simulink model "nested"  (R2020b)
settings: Solver=ode45  StartTime=0.0  StopTime=250  RelTol=1e-3  EnableMultiTasking=on
values from neighbouring files (symbols this model uses):
  apsi1 = 2.374    [Principal.m]
  apsi2 = 0.08    [Principal.m]
  az1 = 3    [Principal.m]
  az2 = 0.5    [Principal.m]
  bphi1 = 2    [Principal.m]
  bphi2 = 1    [Principal.m]
  bphi3 = 0.2    [Principal.m]
  bphi4 = 0.1    [Principal.m]
  bth1 = 2    [Principal.m]
  bth2 = 1    [Principal.m]
  bth3 = 0.2    [Principal.m]
  bth4 = 0.1    [Principal.m]
  ci_phi = 0    [Principal.m]
  ci_phip = 0    [Principal.m]
  ci_psi = 0    [Principal.m]
  ci_psip = 0    [Principal.m]
  ci_th = 0    [Principal.m]
  ci_thp = 0    [Principal.m]
  ci_x = 100    [Principal.m]
  ci_xp = 0    [Principal.m]
  ci_y = 70    [Principal.m]
  ci_yp = 0    [Principal.m]
  ci_z = 0    [Principal.m]
  ci_zp = 0    [Principal.m]
  g = 9.81    [Principal.m]
  m = 0.52    [Principal.m]
  mg = m*g    (= 5.1012)    [Principal.m]
  psid = 0.5    [Principal.m]
  zd = 50    [Principal.m]
libraries: simulink x32
settings Model: Creator=cesar  LastModifiedBy=20808
settings DataIOCC: LimitDataPoints=on  SaveFormat=Array  SignalLoggingSaveFormat=ModelDataLogs  ReturnWorkspaceOutputs=off
settings OptimizationCC: ExpressionDepthLimit=2147483647  InitFltsAndDblsToZero=on  LifeSpan=inf
settings DebuggingCC: UnderspecifiedInitializationDetection=Classic  MergeDetectMultiDrivingBlocksExec=none  SolverPrmCheckMsg=warning  FcnCallInpInsideContextMsg=warning  StateNameClashWarn=warning  SFUnexpectedBacktrackingDiag=warning  SFNoUnconditionalDefaultTransitionDiag=warning  SFExecutionAtInitializationDiag=none  ArithmeticOperatorsInVariantConditions=warning
settings HardwareCC: ProdBitPerPointer=32  ProdBitPerSizeT=32  ProdBitPerPtrDiffT=32  ProdLargestAtomicFloat=None  ProdIntDivRoundTo=Undefined  ProdEndianess=Unspecified  ProdWordSize=32  ProdHWDeviceType=32-bit Generic
settings ModelReferenceCC: PropagateSignalLabelsOutOfModel=off
settings SFSimCC: SimUseLocalCustomCode=off  SimParseCustomCode=off  CustomCodeUndefinedFunction=UseInterfaceOnly
settings RTWCC: RTWUseLocalCustomCode=off
settings CodeAppCC: StateflowObjectComments=on
settings GRTTargetCC: TargetLangStandard=C89/C90 (ANSI)  CombineOutputUpdateFcns=off  GRTInterface=on
settings ConfigComp: CovMetricSettings=dw  CovSaveCumulativeToWorkspaceVar=on  CovSaveSingleToWorkspaceVar=on  CovExternalEMLEnable=off

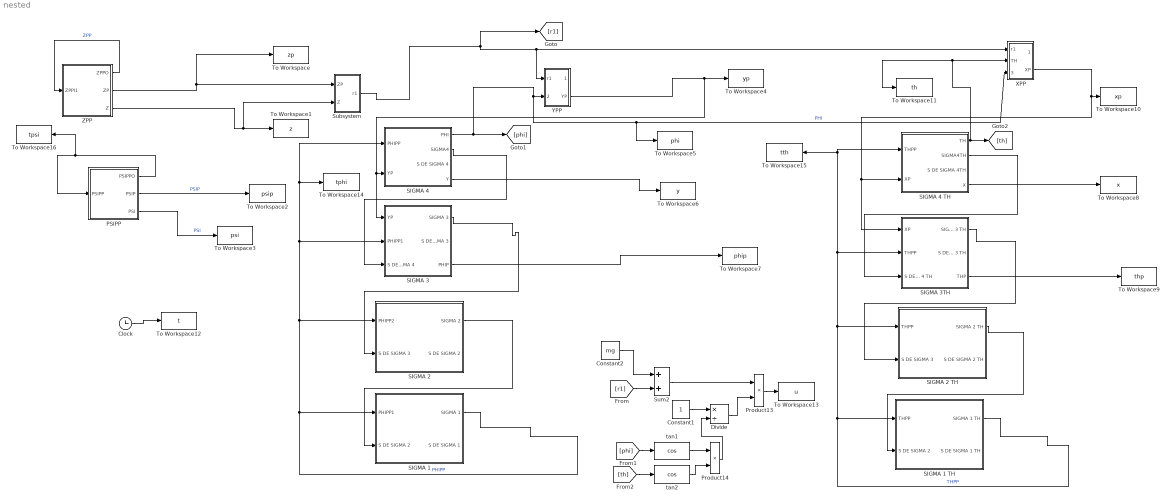
== system nested ==
  Clock : Clock
  Constant1 : Constant
  Constant2 : Constant  Value=mg
  Divide : Product  Inputs=*/
  PSIPP : Subsystem
  Product13 : Product  RndMeth=Zero
  Product14 : Product  RndMeth=Zero
  SIGMA 1 : Subsystem
  SIGMA 1 TH : Subsystem
  SIGMA 2 : Subsystem
  SIGMA 2 TH : Subsystem
  SIGMA 3 : Subsystem
  SIGMA 3TH : Subsystem
  SIGMA 4 : Subsystem
  SIGMA 4 TH : Subsystem
  Subsystem : Subsystem
  Sum2 : Sum
  To Workspace : ToWorkspace  VariableName=zp  SampleTime=-1
  To Workspace1 : ToWorkspace  VariableName=z  SampleTime=-1
  To Workspace10 : ToWorkspace  VariableName=xp  SampleTime=-1
  To Workspace11 : ToWorkspace  VariableName=th  SampleTime=-1
  To Workspace12 : ToWorkspace  VariableName=t  SampleTime=-1
  To Workspace13 : ToWorkspace  VariableName=u  SampleTime=-1
  To Workspace14 : ToWorkspace  VariableName=tphi  SampleTime=-1
  To Workspace15 : ToWorkspace  VariableName=tth  SampleTime=-1
  To Workspace16 : ToWorkspace  VariableName=tpsi  SampleTime=-1
  To Workspace2 : ToWorkspace  VariableName=psip  SampleTime=-1
  To Workspace3 : ToWorkspace  VariableName=psi  SampleTime=-1
  To Workspace4 : ToWorkspace  VariableName=yp  SampleTime=-1
  To Workspace5 : ToWorkspace  VariableName=phi  SampleTime=-1
  To Workspace6 : ToWorkspace  VariableName=y  SampleTime=-1
  To Workspace7 : ToWorkspace  VariableName=phip  SampleTime=-1
  To Workspace8 : ToWorkspace  VariableName=x  SampleTime=-1
  To Workspace9 : ToWorkspace  VariableName=thp  SampleTime=-1
  XPP : Subsystem
  YPP : Subsystem
  ZPP : Subsystem
  tan1 : MATLABFcn  MATLABFcn=cos
  tan2 : MATLABFcn  MATLABFcn=cos
  wires:
  ZPP/1(ZPPO) -> ZPP/1(ZPPI1)  "ZPP"
  PSIPP/1(PSIPPO) -> PSIPP/1(PSIPP), To Workspace16/1
  SIGMA 4/2(SIGMA4) -> SIGMA 3/3(S DE SIGMA 4)
  SIGMA 3/1(SIGMA 3) -> SIGMA 2/2(S DE SIGMA 3)
  SIGMA 2/1(SIGMA 2) -> SIGMA 1/2(S DE SIGMA 2)
  SIGMA 1/1(SIGMA 1) -> SIGMA 1/1(PHIPP1), SIGMA 2/1(PHIPP2), SIGMA 3/2(PHIPP1), SIGMA 4/1(PHIPP), To Workspace14/1  "PHIPP"
  SIGMA 1 TH/1(SIGMA 1 TH) -> SIGMA 1 TH/1(THPP), SIGMA 2 TH/1(THPP), SIGMA 3TH/2(THPP), SIGMA 4 TH/1(THPP), To Workspace15/1  "THPP"
  SIGMA 2 TH/1(SIGMA 2 TH) -> SIGMA 1 TH/2(S DE SIGMA 2)
  SIGMA 3TH/1(SIGMA 3 TH) -> SIGMA 2 TH/2(S DE SIGMA 3)
  SIGMA 4 TH/2(SIGMA4TH) -> SIGMA 3TH/3(S DE SIGMA 4 TH)
  Subsystem/1(r1) -> XPP/1(r1), YPP/1(r1), [r1]
  Clock/1 -> To Workspace12/1
  ZPP/3(Z) -> To Workspace1/1, Subsystem/2(Z)
  SIGMA 4/4(Y) -> To Workspace6/1
  SIGMA 4/1(PHI) -> YPP/2(PHI), XPP/3(PHI), To Workspace5/1, [phi]  "PHI"
  SIGMA 4 TH/4(X) -> To Workspace8/1
  SIGMA 4 TH/1(TH) -> XPP/2(TH), To Workspace11/1, [th]
  PSIPP/3(PSI) -> To Workspace3/1  "PSI"
  PSIPP/2(PSIP) -> To Workspace2/1  "PSIP"
  SIGMA 3/3(PHIP) -> To Workspace7/1
  SIGMA 3TH/3(THP) -> To Workspace9/1
  XPP/2(XP) -> To Workspace10/1, SIGMA 4 TH/2(XP), SIGMA 3TH/1(XP)
  YPP/2(YP) -> To Workspace4/1, SIGMA 4/2(YP), SIGMA 3/1(YP)
  Constant2/1 -> Sum2/1
  [r1] -> Sum2/2
  Sum2/1 -> Product13/1
  tan1/1 -> Product14/1
  tan2/1 -> Product14/2
  [phi] -> tan1/1
  [th] -> tan2/1
  Constant1/1 -> Divide/1
  Product14/1 -> Divide/2
  Divide/1 -> Product13/2
  Product13/1 -> To Workspace13/1
  ZPP/2(ZP) -> Subsystem/1(ZP), To Workspace/1

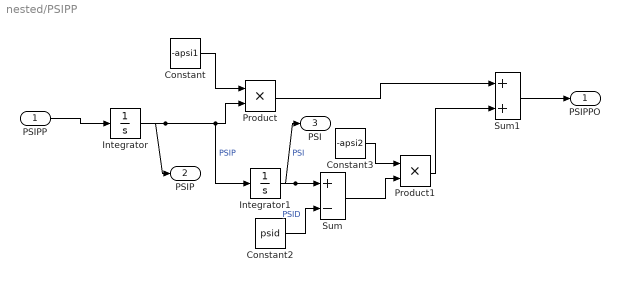
== system nested/PSIPP ==
  PSIPP : Inport
  Constant : Constant  Value=-apsi1
  Constant2 : Constant  Value=psid
  Constant3 : Constant  Value=-apsi2
  Integrator : Integrator  InitialCondition=ci_psip
  Integrator1 : Integrator  InitialCondition=ci_psi
  Product : Product  RndMeth=Zero
  Product1 : Product  RndMeth=Zero
  Sum : Sum  Inputs=+-
  Sum1 : Sum
  PSIPPO : Outport
  PSIP : Outport  Port=2
  PSI : Outport  Port=3
  wires:
  PSIPP/1 -> Integrator/1
  Constant/1 -> Product/1
  Integrator/1 -> Integrator1/1, Product/2, PSIP/1  "PSIP"
  Integrator1/1 -> PSI/1, Sum/1  "PSI"
  Constant2/1 -> Sum/2  "PSID"
  Sum/1 -> Product1/2
  Constant3/1 -> Product1/1
  Product/1 -> Sum1/1
  Product1/1 -> Sum1/2
  Sum1/1 -> PSIPPO/1

== system nested/SIGMA 1 ==
  PHIPP1 : Inport
  S DE SIGMA 2 : Inport  Port=2
  9 : Product  RndMeth=Zero
  Comparador : Subsystem
  Constant2 : Constant  Value=-1  VectorParams1D=off
  Integrator1 : Integrator  InitialCondition=ci_phip
  Sum : Sum  AccumDataTypeStr=double  OutDataTypeStr=double
  SIGMA 1 : Outport
  S DE SIGMA 1 : Outport  Port=2
  wires:
  PHIPP1/1 -> Integrator1/1
  Sum/1 -> S DE SIGMA 1/1, Comparador/1(S DE SIGMA 1)
  Integrator1/1 -> Sum/1  "PHIP"
  S DE SIGMA 2/1 -> Sum/2
  Comparador/1(SIGMA1) -> 9/2
  Constant2/1 -> 9/1
  9/1 -> SIGMA 1/1

== system nested/SIGMA 1 TH ==
  THPP : Inport
  S DE SIGMA 2 : Inport  Port=2
  9 : Product  OutDataTypeStr=double  RndMeth=Zero
  Comparador : Subsystem
  Constant2 : Constant  Value=-1  VectorParams1D=off
  Integrator1 : Integrator  InitialCondition=ci_thp
  Sum : Sum  OutDataTypeStr=double
  SIGMA 1 TH : Outport
  S DE SIGMA 1 TH : Outport  Port=2
  wires:
  S DE SIGMA 2/1 -> Sum/2
  Integrator1/1 -> Sum/1  "THP"
  Sum/1 -> S DE SIGMA 1 TH/1, Comparador/1(S DE SIGMA1 TH)
  THPP/1 -> Integrator1/1
  Comparador/1(SIGMA1TH) -> 9/2
  Constant2/1 -> 9/1
  9/1 -> SIGMA 1 TH/1

== system nested/SIGMA 2 ==
  PHIPP2 : Inport
  S DE SIGMA 3 : Inport  Port=2
  Comparador : Subsystem
  Integrator1 : Integrator  InitialCondition=ci_phip
  Integrator3 : Integrator  InitialCondition=ci_phi
  Sum : Sum  Inputs=+++  InputSameDT=on  AccumDataTypeStr=double  OutDataTypeStr=double
  SIGMA 2 : Outport
  S DE SIGMA 2 : Outport  Port=2
  wires:
  Sum/1 -> S DE SIGMA 2/1, Comparador/1(S DE SIGMA 2)
  PHIPP2/1 -> Integrator1/1
  Integrator3/1 -> Sum/1  "PHI"
  Integrator1/1 -> Integrator3/1, Sum/2  "PHIP"
  S DE SIGMA 3/1 -> Sum/3
  Comparador/1(SIGMA2) -> SIGMA 2/1

== system nested/SIGMA 2 TH ==
  THPP : Inport
  S DE SIGMA 3 : Inport  Port=2
  Comparador : Subsystem
  Integrator1 : Integrator  InitialCondition=ci_thp
  Integrator3 : Integrator  InitialCondition=ci_th
  Sum : Sum  Inputs=+++
  SIGMA 2 TH : Outport
  S DE SIGMA 2 TH : Outport  Port=2
  wires:
  S DE SIGMA 3/1 -> Sum/3
  Integrator1/1 -> Sum/2, Integrator3/1  "THP"
  Integrator3/1 -> Sum/1  "TH"
  THPP/1 -> Integrator1/1
  Sum/1 -> S DE SIGMA 2 TH/1, Comparador/1(S DE SIGMA 2TH)
  Comparador/1(SIGMA2 TH) -> SIGMA 2 TH/1

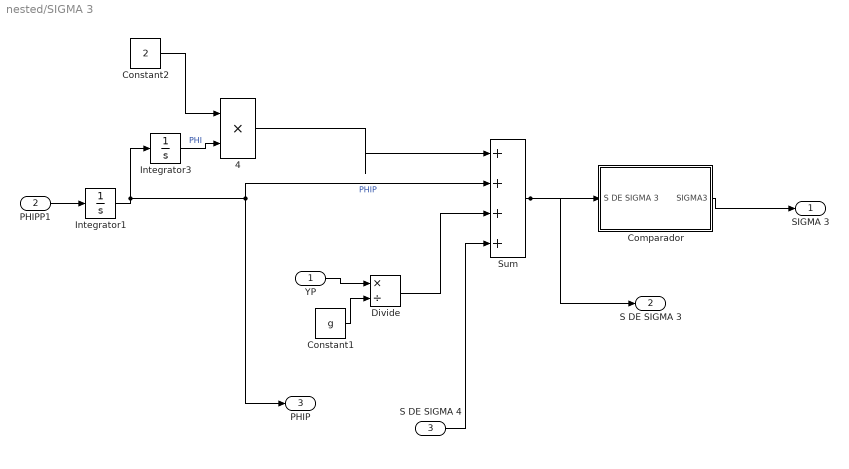
== system nested/SIGMA 3 ==
  YP : Inport
  PHIPP1 : Inport  Port=2
  S DE SIGMA 4 : Inport  Port=3
  4 : Product  RndMeth=Zero
  Comparador : Subsystem
  Constant1 : Constant  Value=g  OutDataTypeStr=double
  Constant2 : Constant  Value=2  OutDataTypeStr=double
  Divide : Product  Inputs=*/
  Integrator1 : Integrator  InitialCondition=ci_phip
  Integrator3 : Integrator  InitialCondition=ci_phi
  Sum : Sum  Inputs=|++++  InputSameDT=on  AccumDataTypeStr=double  OutDataTypeStr=double
  SIGMA 3 : Outport
  S DE SIGMA 3 : Outport  Port=2
  PHIP : Outport  Port=3
  wires:
  Integrator1/1 -> Integrator3/1, Sum/2, PHIP/1  "PHIP"
  Integrator3/1 -> 4/2  "PHI"
  PHIPP1/1 -> Integrator1/1
  Sum/1 -> S DE SIGMA 3/1, Comparador/1(S DE SIGMA 3)
  S DE SIGMA 4/1 -> Sum/4
  Comparador/1(SIGMA3) -> SIGMA 3/1
  YP/1 -> Divide/1
  Constant1/1 -> Divide/2
  Divide/1 -> Sum/3
  4/1 -> Sum/1
  Constant2/1 -> 4/1

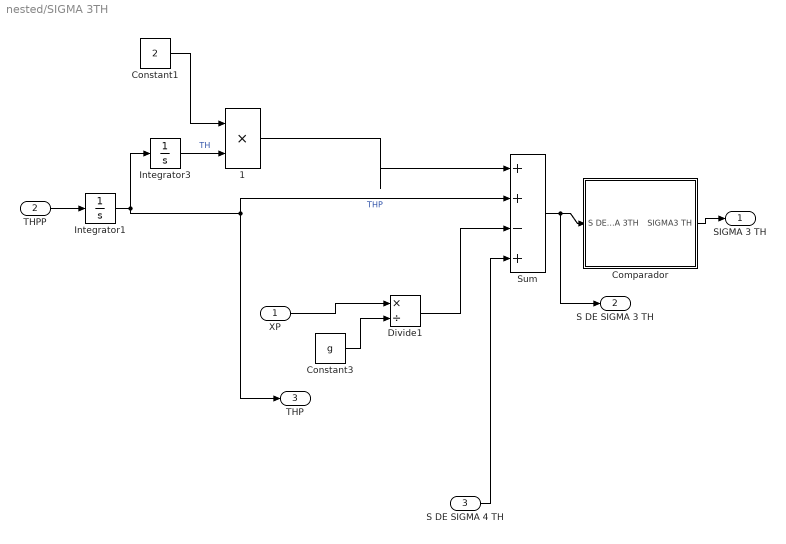
== system nested/SIGMA 3TH ==
  XP : Inport
  THPP : Inport  Port=2
  S DE SIGMA 4 TH : Inport  Port=3
  1 : Product  RndMeth=Zero
  Comparador : Subsystem
  Constant1 : Constant  Value=2  OutDataTypeStr=double
  Constant3 : Constant  Value=g  OutDataTypeStr=double
  Divide1 : Product  Inputs=*/
  Integrator1 : Integrator  InitialCondition=ci_thp
  Integrator3 : Integrator  InitialCondition=ci_th
  Sum : Sum  Inputs=|++-+  OutDataTypeStr=double
  SIGMA 3 TH : Outport
  S DE SIGMA 3 TH : Outport  Port=2
  THP : Outport  Port=3
  wires:
  Sum/1 -> S DE SIGMA 3 TH/1, Comparador/1(S DE SIGMA 3TH)
  THPP/1 -> Integrator1/1
  Integrator1/1 -> Integrator3/1, Sum/2, THP/1  "THP"
  Comparador/1(SIGMA3 TH) -> SIGMA 3 TH/1
  S DE SIGMA 4 TH/1 -> Sum/4
  XP/1 -> Divide1/1
  Constant3/1 -> Divide1/2
  Divide1/1 -> Sum/3
  Integrator3/1 -> 1/2  "TH"
  Constant1/1 -> 1/1
  1/1 -> Sum/1

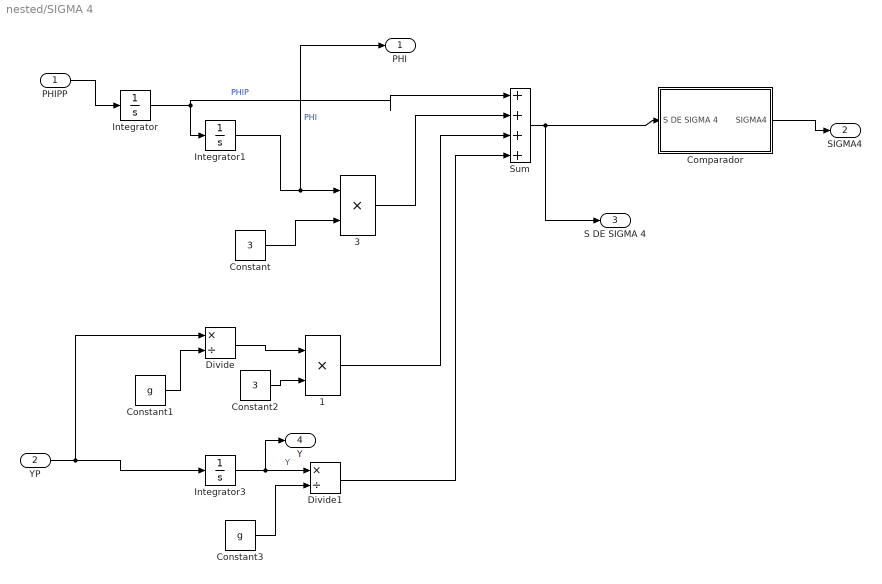
== system nested/SIGMA 4 ==
  PHIPP : Inport
  YP : Inport  Port=2
  1 : Product  RndMeth=Zero
  3 : Product  RndMeth=Zero
  Comparador : Subsystem
  Constant : Constant  Value=3  OutDataTypeStr=double
  Constant1 : Constant  Value=g  OutDataTypeStr=double
  Constant2 : Constant  Value=3  OutDataTypeStr=double
  Constant3 : Constant  Value=g  OutDataTypeStr=double
  Divide : Product  Inputs=*/
  Divide1 : Product  Inputs=*/
  Integrator : Integrator  InitialCondition=ci_phip
  Integrator1 : Integrator  InitialCondition=ci_phi
  Integrator3 : Integrator  InitialCondition=ci_y
  Sum : Sum  Inputs=|++++
  PHI : Outport
  SIGMA4 : Outport  Port=2
  S DE SIGMA 4 : Outport  Port=3
  Y : Outport  Port=4
  wires:
  PHIPP/1 -> Integrator/1
  Integrator/1 -> Integrator1/1, Sum/1  "PHIP"
  3/1 -> Sum/2
  Integrator3/1 -> Divide1/1, Y/1  "Y"
  Divide1/1 -> Sum/4
  Sum/1 -> S DE SIGMA 4/1, Comparador/1(S DE SIGMA 4)
  Comparador/1(SIGMA4) -> SIGMA4/1
  Constant/1 -> 3/2
  Integrator1/1 -> 3/1, PHI/1  "PHI"
  YP/1 -> Divide/1, Integrator3/1
  Constant1/1 -> Divide/2
  Divide/1 -> 1/1
  Constant2/1 -> 1/2
  1/1 -> Sum/3
  Constant3/1 -> Divide1/2

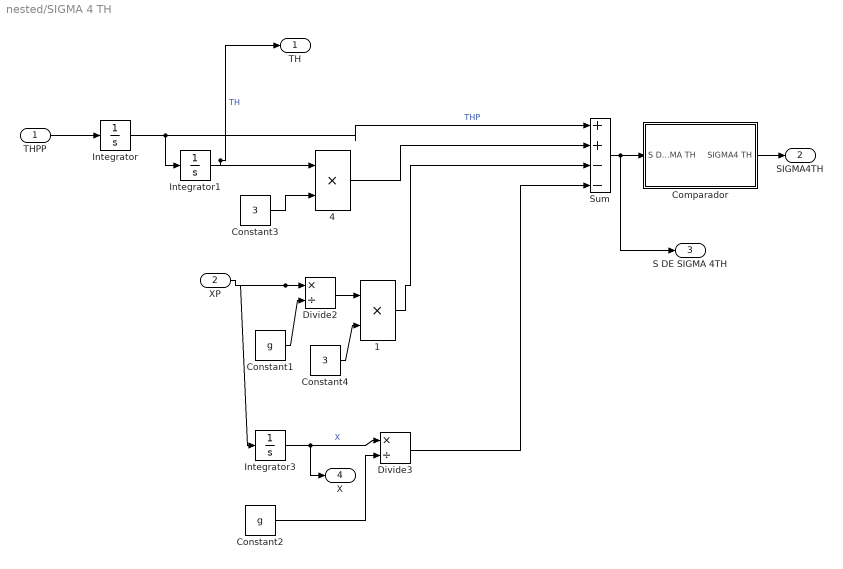
== system nested/SIGMA 4 TH ==
  THPP : Inport
  XP : Inport  Port=2
  1 : Product  RndMeth=Zero
  4 : Product  RndMeth=Zero
  Comparador : Subsystem
  Constant1 : Constant  Value=g  OutDataTypeStr=double
  Constant2 : Constant  Value=g  OutDataTypeStr=double
  Constant3 : Constant  Value=3  OutDataTypeStr=double
  Constant4 : Constant  Value=3  OutDataTypeStr=double
  Divide2 : Product  Inputs=*/
  Divide3 : Product  Inputs=*/
  Integrator : Integrator  InitialCondition=ci_thp
  Integrator1 : Integrator  InitialCondition=ci_th
  Integrator3 : Integrator  InitialCondition=ci_x
  Sum : Sum  Inputs=|++--
  TH : Outport
  SIGMA4TH : Outport  Port=2
  S DE SIGMA 4TH : Outport  Port=3
  X : Outport  Port=4
  wires:
  Sum/1 -> S DE SIGMA 4TH/1, Comparador/1(S DE SIGMA TH)
  1/1 -> Sum/3
  Integrator3/1 -> X/1, Divide3/1  "X"
  XP/1 -> Integrator3/1, Divide2/1
  Integrator1/1 -> TH/1, 4/1  "TH"
  Integrator/1 -> Integrator1/1, Sum/1  "THP"
  THPP/1 -> Integrator/1
  Comparador/1(SIGMA4 TH) -> SIGMA4TH/1
  Constant3/1 -> 4/2
  4/1 -> Sum/2
  Constant1/1 -> Divide2/2
  Divide2/1 -> 1/1
  Constant4/1 -> 1/2
  Constant2/1 -> Divide3/2
  Divide3/1 -> Sum/4

== system nested/Subsystem ==
  ZP : Inport
  Z : Inport  Port=2
  Constant2 : Constant  Value=-az1
  Constant3 : Constant  Value=zd
  Constant4 : Constant  Value=az2
  Product1 : Product  RndMeth=Zero
  Product2 : Product  RndMeth=Zero
  Sum2 : Sum  Inputs=+-
  Sum3 : Sum  Inputs=+-
  r1 : Outport
  wires:
  Constant2/1 -> Product1/1
  Product1/1 -> Sum2/1
  Constant3/1 -> Sum3/2
  Sum3/1 -> Product2/1
  Constant4/1 -> Product2/2
  Product2/1 -> Sum2/2
  Sum2/1 -> r1/1
  ZP/1 -> Product1/2
  Z/1 -> Sum3/1

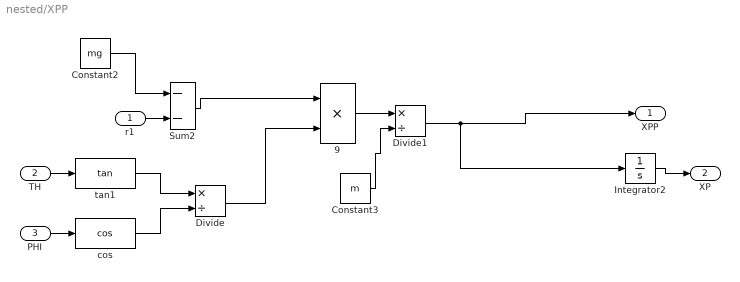
== system nested/XPP ==
  r1 : Inport
  TH : Inport  Port=2
  PHI : Inport  Port=3
  9 : Product  OutDataTypeStr=double  RndMeth=Zero
  Constant2 : Constant  Value=mg
  Constant3 : Constant  Value=m  OutDataTypeStr=double
  Divide : Product  Inputs=*/
  Divide1 : Product  Inputs=*/
  Integrator2 : Integrator  InitialCondition=ci_xp
  Sum2 : Sum  Inputs=--
  cos : MATLABFcn  MATLABFcn=cos
  tan1 : MATLABFcn  MATLABFcn=tan
  XPP : Outport
  XP : Outport  Port=2
  wires:
  Constant2/1 -> Sum2/1
  Sum2/1 -> 9/1
  Integrator2/1 -> XP/1
  r1/1 -> Sum2/2
  TH/1 -> tan1/1
  9/1 -> Divide1/1
  PHI/1 -> cos/1
  tan1/1 -> Divide/1
  cos/1 -> Divide/2
  Divide/1 -> 9/2
  Constant3/1 -> Divide1/2
  Divide1/1 -> XPP/1, Integrator2/1

== system nested/YPP ==
  r1 : Inport
  PHI : Inport  Port=2
  9 : Product  OutDataTypeStr=double  RndMeth=Zero
  Constant2 : Constant  Value=mg
  Constant3 : Constant  Value=m  OutDataTypeStr=double
  Divide1 : Product  Inputs=*/
  Integrator2 : Integrator  InitialCondition=ci_yp
  Sum2 : Sum
  tan1 : MATLABFcn  MATLABFcn=tan
  YPP : Outport
  YP : Outport  Port=2
  wires:
  Constant2/1 -> Sum2/1
  tan1/1 -> 9/2
  Sum2/1 -> 9/1
  Integrator2/1 -> YP/1
  r1/1 -> Sum2/2
  PHI/1 -> tan1/1
  9/1 -> Divide1/1
  Constant3/1 -> Divide1/2
  Divide1/1 -> YPP/1, Integrator2/1

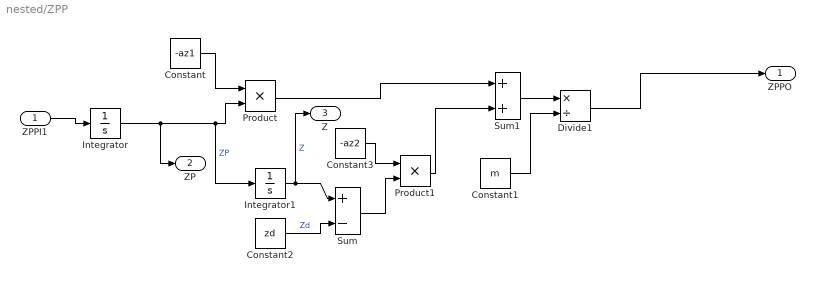
== system nested/ZPP ==
  ZPPI1 : Inport
  Constant : Constant  Value=-az1
  Constant1 : Constant  Value=m
  Constant2 : Constant  Value=zd
  Constant3 : Constant  Value=-az2
  Divide1 : Product  Inputs=*/
  Integrator : Integrator  InitialCondition=ci_zp
  Integrator1 : Integrator  InitialCondition=ci_z
  Product : Product  RndMeth=Zero
  Product1 : Product  RndMeth=Zero
  Sum : Sum  Inputs=+-
  Sum1 : Sum
  ZPPO : Outport
  ZP : Outport  Port=2
  Z : Outport  Port=3
  wires:
  Product1/1 -> Sum1/2
  Product/1 -> Sum1/1
  Constant3/1 -> Product1/1
  Sum/1 -> Product1/2
  Constant2/1 -> Sum/2  "Zd"
  Integrator1/1 -> Sum/1, Z/1  "Z"
  Integrator/1 -> Product/2, Integrator1/1, ZP/1  "ZP"
  Constant/1 -> Product/1
  Divide1/1 -> ZPPO/1
  ZPPI1/1 -> Integrator/1
  Sum1/1 -> Divide1/1
  Constant1/1 -> Divide1/2

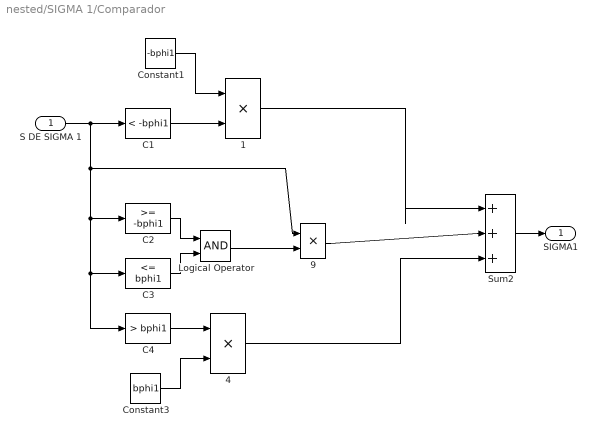
== system nested/SIGMA 1/Comparador ==
  S DE SIGMA 1 : Inport
  1 : Product  RndMeth=Zero
  4 : Product  RndMeth=Zero
  9 : Product  RndMeth=Zero
  C1 : simulink/Logic and Bit Operations/Compare To Constant  relop=<  const=-bphi1  OutDataTypeStr=boolean  ZeroCross=off
  C2 : simulink/Logic and Bit Operations/Compare To Constant  relop=>=  const=-bphi1  OutDataTypeStr=boolean  ZeroCross=off
  C3 : simulink/Logic and Bit Operations/Compare To Constant  relop=<=  const=bphi1  OutDataTypeStr=boolean  ZeroCross=off
  C4 : simulink/Logic and Bit Operations/Compare To Constant  relop=>  const=bphi1  OutDataTypeStr=boolean  ZeroCross=off
  Constant1 : Constant  Value=-bphi1  OutDataTypeStr=double
  Constant3 : Constant  Value=bphi1  OutDataTypeStr=double
  Logical Operator : Logic  AllPortsSameDT=off  OutDataTypeStr=boolean
  Sum2 : Sum  Inputs=|+++
  SIGMA1 : Outport
  wires:
  S DE SIGMA 1/1 -> C1/1, C2/1, C3/1, C4/1, 9/1
  C1/1 -> 1/2
  C2/1 -> Logical Operator/1
  C3/1 -> Logical Operator/2
  Logical Operator/1 -> 9/2
  C4/1 -> 4/1
  9/1 -> Sum2/2
  Sum2/1 -> SIGMA1/1
  Constant3/1 -> 4/2
  4/1 -> Sum2/3
  Constant1/1 -> 1/1
  1/1 -> Sum2/1

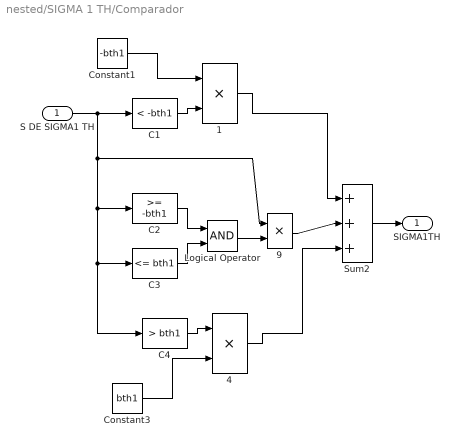
== system nested/SIGMA 1 TH/Comparador ==
  S DE SIGMA1 TH : Inport
  1 : Product  RndMeth=Zero
  4 : Product  RndMeth=Zero
  9 : Product  OutDataTypeStr=double  RndMeth=Zero
  C1 : simulink/Logic and Bit Operations/Compare To Constant  relop=<  const=-bth1  OutDataTypeStr=boolean  ZeroCross=off
  C2 : simulink/Logic and Bit Operations/Compare To Constant  relop=>=  const=-bth1  OutDataTypeStr=boolean  ZeroCross=off
  C3 : simulink/Logic and Bit Operations/Compare To Constant  relop=<=  const=bth1  OutDataTypeStr=boolean  ZeroCross=off
  C4 : simulink/Logic and Bit Operations/Compare To Constant  relop=>  const=bth1  OutDataTypeStr=boolean  ZeroCross=off
  Constant1 : Constant  Value=-bth1  OutDataTypeStr=double
  Constant3 : Constant  Value=bth1  OutDataTypeStr=double
  Logical Operator : Logic  AllPortsSameDT=off  OutDataTypeStr=boolean
  Sum2 : Sum  Inputs=|+++  OutDataTypeStr=double
  SIGMA1TH : Outport
  wires:
  S DE SIGMA1 TH/1 -> C1/1, C2/1, C3/1, C4/1, 9/1
  C1/1 -> 1/2
  C2/1 -> Logical Operator/1
  C3/1 -> Logical Operator/2
  Logical Operator/1 -> 9/2
  C4/1 -> 4/1
  1/1 -> Sum2/1
  9/1 -> Sum2/2
  4/1 -> Sum2/3
  Sum2/1 -> SIGMA1TH/1
  Constant3/1 -> 4/2
  Constant1/1 -> 1/1

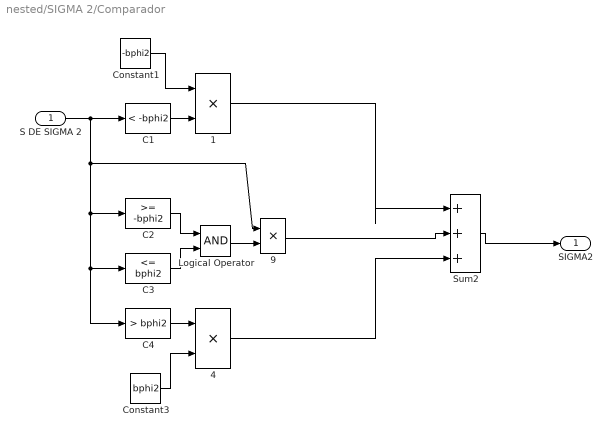
== system nested/SIGMA 2/Comparador ==
  S DE SIGMA 2 : Inport
  1 : Product  RndMeth=Zero
  4 : Product  RndMeth=Zero
  9 : Product  RndMeth=Zero
  C1 : simulink/Logic and Bit Operations/Compare To Constant  relop=<  const=-bphi2  OutDataTypeStr=boolean  ZeroCross=off
  C2 : simulink/Logic and Bit Operations/Compare To Constant  relop=>=  const=-bphi2  OutDataTypeStr=boolean  ZeroCross=off
  C3 : simulink/Logic and Bit Operations/Compare To Constant  relop=<=  const=bphi2  OutDataTypeStr=boolean  ZeroCross=off
  C4 : simulink/Logic and Bit Operations/Compare To Constant  relop=>  const=bphi2  OutDataTypeStr=boolean  ZeroCross=off
  Constant1 : Constant  Value=-bphi2  OutDataTypeStr=double
  Constant3 : Constant  Value=bphi2  OutDataTypeStr=double
  Logical Operator : Logic  AllPortsSameDT=off  OutDataTypeStr=boolean
  Sum2 : Sum  Inputs=|+++
  SIGMA2 : Outport
  wires:
  S DE SIGMA 2/1 -> C1/1, C2/1, C3/1, C4/1, 9/1
  C1/1 -> 1/2
  C2/1 -> Logical Operator/1
  C3/1 -> Logical Operator/2
  Logical Operator/1 -> 9/2
  C4/1 -> 4/1
  9/1 -> Sum2/2
  Sum2/1 -> SIGMA2/1
  Constant3/1 -> 4/2
  4/1 -> Sum2/3
  Constant1/1 -> 1/1
  1/1 -> Sum2/1

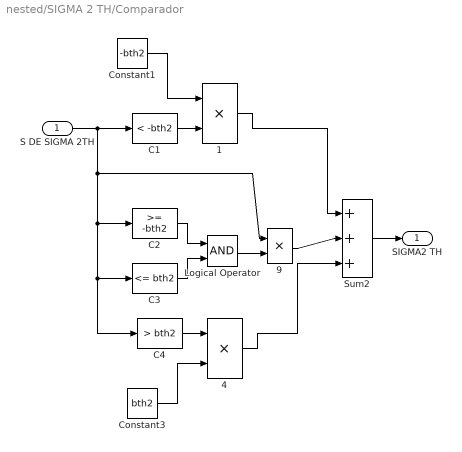
== system nested/SIGMA 2 TH/Comparador ==
  S DE SIGMA 2TH : Inport
  1 : Product  RndMeth=Zero
  4 : Product  RndMeth=Zero
  9 : Product  OutDataTypeStr=double  RndMeth=Zero
  C1 : simulink/Logic and Bit Operations/Compare To Constant  relop=<  const=-bth2  OutDataTypeStr=boolean  ZeroCross=off
  C2 : simulink/Logic and Bit Operations/Compare To Constant  relop=>=  const=-bth2  OutDataTypeStr=boolean  ZeroCross=off
  C3 : simulink/Logic and Bit Operations/Compare To Constant  relop=<=  const=bth2  OutDataTypeStr=boolean  ZeroCross=off
  C4 : simulink/Logic and Bit Operations/Compare To Constant  relop=>  const=bth2  OutDataTypeStr=boolean  ZeroCross=off
  Constant1 : Constant  Value=-bth2  OutDataTypeStr=double
  Constant3 : Constant  Value=bth2  OutDataTypeStr=double
  Logical Operator : Logic  AllPortsSameDT=off  OutDataTypeStr=boolean
  Sum2 : Sum  Inputs=|+++  OutDataTypeStr=double
  SIGMA2 TH : Outport
  wires:
  S DE SIGMA 2TH/1 -> C1/1, C2/1, C3/1, C4/1, 9/1
  C1/1 -> 1/2
  C2/1 -> Logical Operator/1
  C3/1 -> Logical Operator/2
  Logical Operator/1 -> 9/2
  C4/1 -> 4/1
  1/1 -> Sum2/1
  9/1 -> Sum2/2
  4/1 -> Sum2/3
  Sum2/1 -> SIGMA2 TH/1
  Constant3/1 -> 4/2
  Constant1/1 -> 1/1

== system nested/SIGMA 3/Comparador ==
  S DE SIGMA 3 : Inport
  1 : Product  RndMeth=Zero
  4 : Product  RndMeth=Zero
  9 : Product  RndMeth=Zero
  C1 : simulink/Logic and Bit Operations/Compare To Constant  relop=<  const=-bphi3  OutDataTypeStr=boolean  ZeroCross=off
  C2 : simulink/Logic and Bit Operations/Compare To Constant  relop=>=  const=-bphi3  OutDataTypeStr=boolean  ZeroCross=off
  C3 : simulink/Logic and Bit Operations/Compare To Constant  relop=<=  const=bphi3  OutDataTypeStr=boolean  ZeroCross=off
  C4 : simulink/Logic and Bit Operations/Compare To Constant  relop=>  const=bphi3  OutDataTypeStr=boolean  ZeroCross=off
  Constant1 : Constant  Value=-bphi3  OutDataTypeStr=double
  Constant3 : Constant  Value=bphi3  OutDataTypeStr=double
  Logical Operator : Logic  AllPortsSameDT=off  OutDataTypeStr=boolean
  Sum2 : Sum  Inputs=|+++
  SIGMA3 : Outport
  wires:
  S DE SIGMA 3/1 -> C1/1, C2/1, C3/1, C4/1, 9/1
  C1/1 -> 1/2
  C2/1 -> Logical Operator/1
  C3/1 -> Logical Operator/2
  Logical Operator/1 -> 9/2
  C4/1 -> 4/1
  1/1 -> Sum2/1
  9/1 -> Sum2/2
  Sum2/1 -> SIGMA3/1
  Constant3/1 -> 4/2
  4/1 -> Sum2/3
  Constant1/1 -> 1/1

== system nested/SIGMA 3TH/Comparador ==
  S DE SIGMA 3TH : Inport
  1 : Product  RndMeth=Zero
  4 : Product  RndMeth=Zero
  9 : Product  OutDataTypeStr=double  RndMeth=Zero
  C1 : simulink/Logic and Bit Operations/Compare To Constant  relop=<  const=-bth3  OutDataTypeStr=boolean  ZeroCross=off
  C2 : simulink/Logic and Bit Operations/Compare To Constant  relop=>=  const=-bth3  OutDataTypeStr=boolean  ZeroCross=off
  C3 : simulink/Logic and Bit Operations/Compare To Constant  relop=<=  const=bth3  OutDataTypeStr=boolean  ZeroCross=off
  C4 : simulink/Logic and Bit Operations/Compare To Constant  relop=>  const=bth3  OutDataTypeStr=boolean  ZeroCross=off
  Constant1 : Constant  Value=-bth3  OutDataTypeStr=double
  Constant3 : Constant  Value=bth3  OutDataTypeStr=double
  Logical Operator : Logic  AllPortsSameDT=off  OutDataTypeStr=boolean
  Sum2 : Sum  Inputs=|+++  OutDataTypeStr=double
  SIGMA3 TH : Outport
  wires:
  S DE SIGMA 3TH/1 -> C1/1, C2/1, C3/1, C4/1, 9/1
  C1/1 -> 1/2
  C2/1 -> Logical Operator/1
  C3/1 -> Logical Operator/2
  Logical Operator/1 -> 9/2
  C4/1 -> 4/1
  9/1 -> Sum2/2
  4/1 -> Sum2/3
  Sum2/1 -> SIGMA3 TH/1
  Constant3/1 -> 4/2
  Constant1/1 -> 1/1
  1/1 -> Sum2/1

== system nested/SIGMA 4/Comparador ==
  S DE SIGMA 4 : Inport
  1 : Product  OutDataTypeStr=double  RndMeth=Zero
  2 : Product  OutDataTypeStr=double  RndMeth=Zero
  9 : Product  OutDataTypeStr=double  RndMeth=Zero
  C1 : simulink/Logic and Bit Operations/Compare To Constant  relop=<  const=-bphi4  OutDataTypeStr=boolean  ZeroCross=off
  C2 : simulink/Logic and Bit Operations/Compare To Constant  relop=>=  const=-bphi4  OutDataTypeStr=boolean  ZeroCross=off
  C3 : simulink/Logic and Bit Operations/Compare To Constant  relop=<=  const=bphi4  OutDataTypeStr=boolean  ZeroCross=off
  C4 : simulink/Logic and Bit Operations/Compare To Constant  relop=>  const=bphi4  OutDataTypeStr=boolean  ZeroCross=off
  Constant1 : Constant  Value=bphi4  OutDataTypeStr=double
  Constant2 : Constant  Value=-bphi4  OutDataTypeStr=double
  Logical Operator : Logic  AllPortsSameDT=off  OutDataTypeStr=boolean
  Sum2 : Sum  Inputs=|+++
  SIGMA4 : Outport
  wires:
  S DE SIGMA 4/1 -> C1/1, C2/1, C3/1, C4/1, 9/1
  C1/1 -> 1/2
  C2/1 -> Logical Operator/1
  C3/1 -> Logical Operator/2
  Logical Operator/1 -> 9/2
  C4/1 -> 2/1
  1/1 -> Sum2/1
  9/1 -> Sum2/2
  2/1 -> Sum2/3
  Sum2/1 -> SIGMA4/1
  Constant2/1 -> 1/1
  Constant1/1 -> 2/2

== system nested/SIGMA 4 TH/Comparador ==
  S DE SIGMA TH : Inport
  1 : Product  RndMeth=Zero
  4 : Product  RndMeth=Zero
  9 : Product  RndMeth=Zero
  C1 : simulink/Logic and Bit Operations/Compare To Constant  relop=<  const=-bth4  OutDataTypeStr=boolean  ZeroCross=off
  C2 : simulink/Logic and Bit Operations/Compare To Constant  relop=>=  const=-bth4  OutDataTypeStr=boolean  ZeroCross=off
  C3 : simulink/Logic and Bit Operations/Compare To Constant  relop=<=  const=bth4  OutDataTypeStr=boolean  ZeroCross=off
  C4 : simulink/Logic and Bit Operations/Compare To Constant  relop=>  const=bth4  OutDataTypeStr=boolean  ZeroCross=off
  Constant1 : Constant  Value=-bth4  OutDataTypeStr=double
  Constant3 : Constant  Value=bth4  OutDataTypeStr=double
  Logical Operator : Logic  AllPortsSameDT=off  OutDataTypeStr=boolean
  Sum2 : Sum  Inputs=|+++
  SIGMA4 TH : Outport
  wires:
  S DE SIGMA TH/1 -> C1/1, C2/1, C3/1, C4/1, 9/1
  C1/1 -> 1/2
  C2/1 -> Logical Operator/1
  C3/1 -> Logical Operator/2
  Logical Operator/1 -> 9/2
  C4/1 -> 4/1
  1/1 -> Sum2/1
  9/1 -> Sum2/2
  4/1 -> Sum2/3
  Sum2/1 -> SIGMA4 TH/1
  Constant3/1 -> 4/2
  Constant1/1 -> 1/1
